simulink model "abs_quarter_car"  (R2025a)
settings: Solver=ode4  StartTime=0.0  StopTime=5.0  FixedStep=0.0005  RelTol=1e-3
settings Model: Creator=ZORO  LastModifiedBy=ZORO

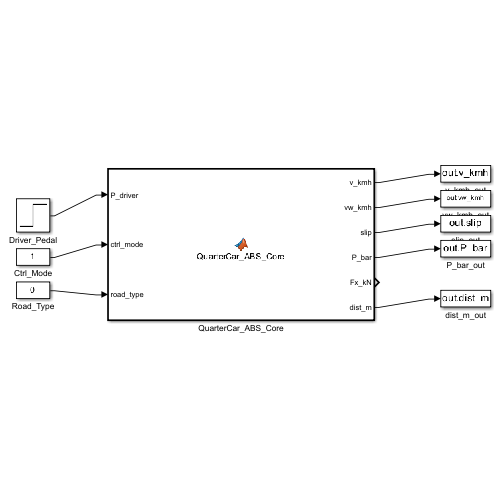
[thumbnail: Simulink's stored preview of the top-level diagram]
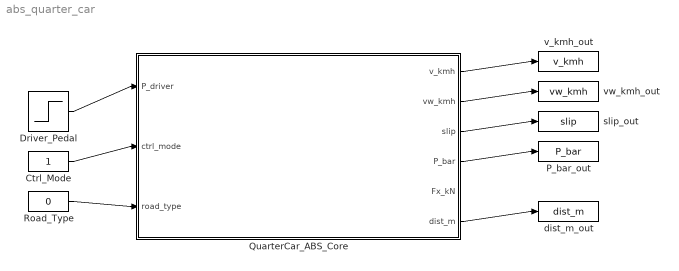
== system abs_quarter_car ==
  Ctrl_Mode : Constant
  Driver_Pedal : Step  Time=0.10  Before=0.0  After=15.0e6  SampleTime=0
  P_bar_out : ToWorkspace  VariableName=P_bar  SampleTime=-1
  QuarterCar_ABS_Core : MATLAB Function  TreatAsAtomicUnit=on
  Road_Type : Constant  Value=0
  dist_m_out : ToWorkspace  VariableName=dist_m  SampleTime=-1
  slip_out : ToWorkspace  VariableName=slip  SampleTime=-1
  v_kmh_out : ToWorkspace  VariableName=v_kmh  SampleTime=-1
  vw_kmh_out : ToWorkspace  VariableName=vw_kmh  SampleTime=-1
  wires:
  Driver_Pedal/1 -> QuarterCar_ABS_Core/1(P_driver)
  Ctrl_Mode/1 -> QuarterCar_ABS_Core/2(ctrl_mode)
  Road_Type/1 -> QuarterCar_ABS_Core/3(road_type)
  QuarterCar_ABS_Core/1(v_kmh) -> v_kmh_out/1
  QuarterCar_ABS_Core/2(vw_kmh) -> vw_kmh_out/1
  QuarterCar_ABS_Core/3(slip) -> slip_out/1
  QuarterCar_ABS_Core/4(P_bar) -> P_bar_out/1
  QuarterCar_ABS_Core/6(dist_m) -> dist_m_out/1

== matlab function abs_quarter_car/QuarterCar_ABS_Core ==
  data: P_driver input; v_kmh output; ctrl_mode input; road_type input; vw_kmh output; slip output; P_bar output; Fx_kN output; dist_m output
function [v_kmh, vw_kmh, slip, P_bar, Fx_kN, dist_m] = QuarterCar_ABS_Core(P_driver, ctrl_mode, road_type)
% Quarter-Car ABS Core Dynamic Simulation Block
% States maintained persistently
persistent v w x P ctrl_phase P_hold w_prev t_last
if isempty(v)
    v = 100 / 3.6; % 100 km/h default initial
    w = v / 0.32;
    x = 0.0;
    P = 0.0;
    ctrl_phase = 0;
    P_hold = 0.0;
    w_prev = w;
    t_last = 0.0;
end

dt = 0.0005;
m  = 400.0;
R  = 0.32;
Jw = 1.20;
g  = 9.81;
Fz = m * g;
Kb = 1.8e-4;

vw = w * R;
slip = (v - vw) / max(v, 0.1);
slip = max(0.0, min(1.0, slip));

% Wheel acceleration
aw = ((w - w_prev) / dt) * R;
w_prev = w;

% Controller Execution
% Mode 0: No ABS | Mode 1: Rule-Based | Mode 2: PID | Mode 3: SMC
if ctrl_mode == 0 || v < 1.5
    P_cmd = P_driver;
elseif ctrl_mode == 1
    % Rule-Based ABS
    is_locking = (slip > 0.19) || (slip > 0.09 && aw < -25.0);
    if ctrl_phase == 0 && is_locking
        ctrl_phase = 2;
        P_hold = 0.78 * P;
    elseif ctrl_phase == 2 && (aw > 3.0 || (slip < 0.15 && aw > 0))
        ctrl_phase = 1;
    elseif ctrl_phase == 1 && (aw < 1.5 && slip < 0.14)
        ctrl_phase = 0;
    end
    if ctrl_phase == 2
        P_cmd = max(0.72 * P_hold, P - 9.0e7 * dt);
    elseif ctrl_phase == 1
        P_cmd = P_hold;
    else
        P_cmd = min(P_driver, P + 8.5e7 * dt);
    end
else
    % PID / SMC closed-loop slip regulation
    target_slip = 0.16;
    e = target_slip - slip;
    P_cmd = max(0.0, min(P_driver, 6.5e6 + 4.5e7 * e));
end

% Actuator lag & rate limit
tau = 0.025;
dP = (P_cmd - P) / tau;
dP = max(-1.2e8, min(8.0e7, dP));
P  = max(0.0, min(15.0e6, P + dP * dt));
Tb = Kb * P;

% Pacejka Friction (Dry Asphalt: B=10, C=1.60, D=1.00, E=0.40)
if road_type == 1 % Wet
    B=12.0; C=1.55; D=0.75; E=0.30;
elseif road_type == 2 % Snow
    B=15.0; C=1.50; D=0.30; E=0.20;
elseif road_type == 3 % Ice
    B=20.0; C=1.45; D=0.15; E=0.10;
else % Dry
    B=10.0; C=1.60; D=1.00; E=0.40;
end
arg = B*slip - E*(B*slip - atan(B*slip));
mu = max(0.0, D * sin(C * atan(arg)));
Fx = mu * Fz;

% Dynamic Integration
if v > 0.5
    v = max(0.0, v - (Fx / m) * dt);
    w = max(0.0, w + ((-Tb + Fx * R) / Jw) * dt);
    x = x + v * dt;
else
    v = 0.0; w = 0.0; Fx = 0.0; Tb = 0.0;
end

v_kmh  = v * 3.6;
vw_kmh = vw * 3.6;
P_bar  = P * 1e-5;
Fx_kN  = Fx * 1e-3;
dist_m = x;
